simulink model "WaterTankSysControlPID2024"  (R2023b)
settings: Solver=FixedStepAuto  StartTime=0.0  StopTime=525  FixedStep=0.75  RelTol=1e-3  EnableMultiTasking=on
StopFcn:
  | FileName='PIDControlData0.mat';
  | [fPath, fName, fExt] = fileparts(FileName);
  | if isempty(fExt)  % No '.mat' in FileName
  |     fExt     = '.mat';
  |     FileName = fullfile(fPath, [fName, fExt]);
  | end
  | if exist(FileName, 'file')
  |     % Get number of files:
  |     fDir     = dir(fullfile(fPath, [fName, '*', fExt]));
  |     fStr     = lower(sprintf('%s*', fDir.name));
  |     %fNum     = sscanf(fStr, [fName, '%d', fExt, '*']);
  |     digit =  str2double(extract(fStr, digitsPattern));
  |     %newNum = digit + 1;
  |     if isempty(digit)
  |         newNum = 1;
  |     else
  |         newNum = digit + 1;
  |     end
  |     FileName = fullfile(fPath, [fName, sprintf('%d', newNum(end)), fExt]);
  | end
  | save(FileName, 'ScopeData1');
  | clear digit fDir fExt FileName fName fPath fStr newNum fNum
values from neighbouring files (symbols this model uses):
  u_offset = u_act(1)    [Lab5.m]
  y_offset = mean(y_act(1:i))    [Lab5.m]
undefined symbols (not defined in the file or in its folder): National_Instruments, PCIe
libraries: sldrtlib x4, slpidlib x1, simulink x1
settings Model: SimulationMode=external  ExtModeTrigDuration=7200  ExtModeArchiveMode=auto  ExtModeArchiveFileName=SysIdenData  ExtModeArchiveDirName=C:\Users\My Project\Documents\MATLAB  ExtModeAutoIncOneShot=on  ExtModeWriteAllDataToWs=on  Creator=My Project  LastModifiedBy=My Project
settings SolverCC: AlgebraicLoopSolver=TrustRegion
settings DataIOCC: LimitDataPoints=on  ReturnWorkspaceOutputs=off
settings OptimizationCC: ReuseModelBlockBuffer=off  LifeSpan=inf
settings DebuggingCC: UnconnectedInputMsg=warning  UnconnectedOutputMsg=warning  UnconnectedLineMsg=warning  AllowSymbolicDim=off  SFUnexpectedBacktrackingDiag=warning  SFNoUnconditionalDefaultTransitionDiag=warning  SFExecutionAtInitializationDiag=none  ArithmeticOperatorsInVariantConditions=warning
settings HardwareCC: ProdBitPerLong=64  ProdHWDeviceType=Intel->x86-64 (Linux 64)  TargetBitPerLong=64  TargetBitPerPointer=64  TargetIntDivRoundTo=Zero  TargetEndianess=LittleEndian  TargetWordSize=64  TargetHWDeviceType=Intel->x86-64
settings ModelReferenceCC: EnableRefExpFcnMdlSchedulingChecks=on  PropagateSignalLabelsOutOfModel=off
settings SFSimCC: SimUseLocalCustomCode=off  CustomCodeUndefinedFunction=UseInterfaceOnly
settings RTWCC: Description=Simulink Desktop Real-Time  SystemTargetFile=sldrt.tlc  TemplateMakefile=sldrt.tmf  RTWUseLocalCustomCode=off  RTWCompilerOptimization=on
settings CodeAppCC: MaxIdLength=95  StateflowObjectComments=on
settings SimulinkDesktopRealTimeCC: TargetLibSuffix=_sldrt.a  TargetPreCompLibLocation=C:\Program Files\MATLAB\R2023b\toolbox\sldrt\lib\win64  TargetLangStandard=C89/C90 (ANSI)  SupportVariableSizeSignals=off
settings ConfigComp: CovMetricSettings=dw  CovSaveCumulativeToWorkspaceVar=on  CovSaveSingleToWorkspaceVar=on  CovExternalEMLEnable=off

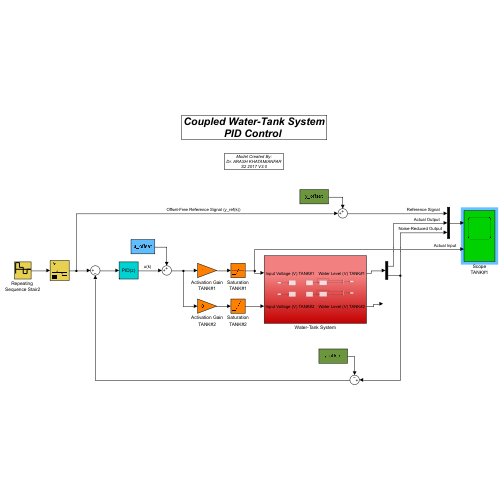
[thumbnail: Simulink's stored preview of the top-level diagram]
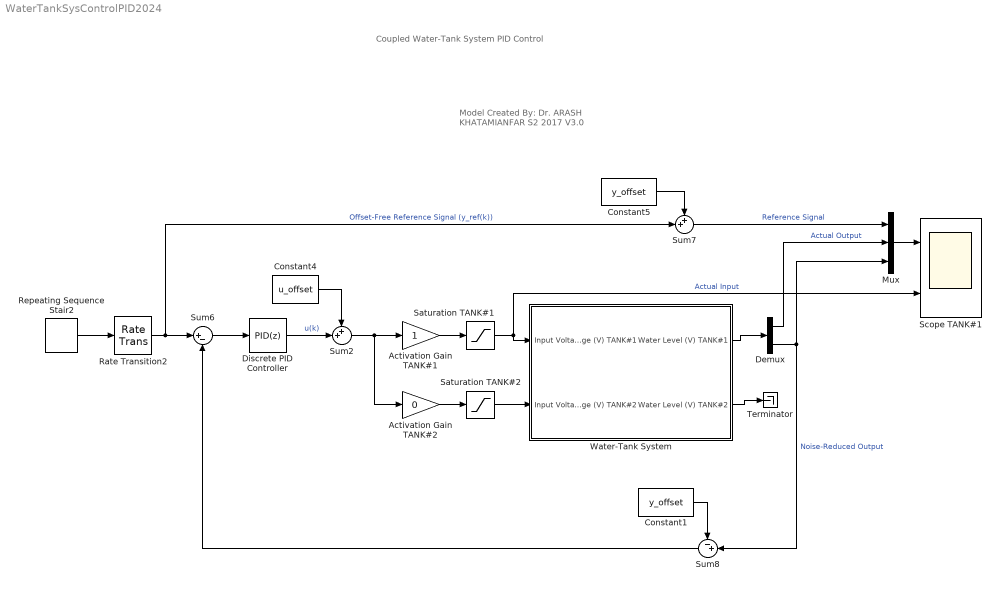
== system WaterTankSysControlPID2024 ==
  note: Model Created By:
      | Dr. ARASH KHATAMIANFAR
      | S2 2017 V3.0
  note: Coupled Water-Tank System
      | PID Control
  Activation Gain TANK#1 : Gain
  Activation Gain TANK#2 : Gain  Gain=0
  Constant1 : Constant  Value=y_offset
  Constant4 : Constant  Value=u_offset
  Constant5 : Constant  Value=y_offset
  Demux : Demux  Outputs=2
  Discrete PID Controller : slpidlib/PID Controller  Controller=PID  Form=Parallel  TimeDomain=Discrete-time  UseExternalTs=off  SampleTime=0.75  IntegratorMethod=Forward Euler  FilterMethod=Forward Euler  ControllerParametersSource=internal  P=0.56  I=0.029  UseKiTs=off  D=0  N=100  UseFilter=on  TunerSelectOption=Transfer Function Based (PID Tuner App)  InitialConditionSource=internal  InitialConditionForIntegrator=0  InitialConditionForFilter=0  DifferentiatorICPrevScaledInput=0  ExternalReset=none  TrackingMode=off  Kt=1  LimitOutput=off  SatLimitsSource=internal  UpperSaturationLimit=inf  LowerSaturationLimit=-inf  LinearizeAsGain=off  AntiWindupMode=none  Kb=1  LimitIntegrator=off  UpperIntegratorSaturationLimit=1  LowerIntegratorSaturationLimit=-1  POutMin=[]  POutMax=[]  IOutMin=[]  IOutMax=[]  DOutMin=[]  DOutMax=[]  NOutMin=[]  NOutMax=[]  SumOutMin=[]  SumOutMax=[]  SaturationOutMin=[]  SaturationOutMax=[]  PParamMin=[]  PParamMax=[]  IParamMin=[]  IParamMax=[]  DParamMin=[]  DParamMax=[]  NParamMin=[]  NParamMax=[]  KbParamMin=[]  KbParamMax=[]  KtParamMin=[]  KtParamMax=[]  KbOutMin=[]  KbOutMax=[]  KtOutMin=[]  KtOutMax=[]  IntegratorOutMin=[]  IntegratorOutMax=[]  FilterOutMin=[]  FilterOutMax=[]  SumI1OutMin=[]  SumI1OutMax=[]  SumI2OutMin=[]  SumI2OutMax=[]  SumI3OutMin=[]  SumI3OutMax=[]  SumI4OutMin=[]  SumI4OutMax=[]  SumDOutMin=[]  SumDOutMax=[]  DifferentiatorOutMin=[]  DifferentiatorOutMax=[]  FilterDiffOutCoefMin=[]  FilterDiffOutCoefMax=[]  ReciprocalOutMin=[]  ReciprocalOutMax=[]  SumDenOutMin=[]  SumDenOutMax=[]  SumNumOutMin=[]  SumNumOutMax=[]  DivideOutMin=[]  DivideOutMax=[]  UdiffTsProdOutMin=[]  UdiffTsProdOutMax=[]  NTsProdOutMin=[]  NTsProdOutMax=[]  UintegralTsProdOutMin=[]  UintegralTsProdOutMax=[]  UngainTsProdOutMin=[]  UngainTsProdOutMax=[]  ClampingZeroOutDataTypeStr=Inherit: Inherit via back propagation  ClampingZeroOutMin=[]  ClampingZeroOutMax=[]  FilterDenConstantOutDataTypeStr=Inherit: Inherit via back propagation  FilterDenConstantOutMin=[]  FilterDenConstantOutMax=[]  PCopyOutDataTypeStr=Inherit: Inherit via back propagation  PCopyOutMin=[]  PCopyOutMax=[]  NCopyOutDataTypeStr=Inherit: Inherit via back propagation  NCopyOutMin=[]  NCopyOutMax=[]  IntegratorContinuousStateAttributes=''  IntegratorStateMustResolveToSignalObject=off  IntegratorRTWStateStorageClass=Auto  FilterContinuousStateAttributes=''  FilterStateMustResolveToSignalObject=off  FilterRTWStateStorageClass=Auto  ParallelPVariant=InternalParameters  IdealPVariant=Disabled  IVariant=InternalParameters  DVariant=InternalParameters  IntegratorVariant=Discrete  SatVariant=Disabled  AWVariant=Passthrough  PCopyVariant=Disabled  TRVariant=Disabled  FdbkBlocksVariant=Forward  IdealPFdbkVariant=Disabled  SatFdbkVariant=Disabled  DerivativeFilterVariant=ForwardEulerFilter  NVariant=InternalParameters  NCopyVariant=Disabled  FilterICVariant=InternalICsFilter  IntegratorICVariant=InternalICs  ExternalResetVariant=Disabled  TRSumVariant=Passthrough  SumFdbkVariant=Disabled  SumVariant=Sum_PID  TsampFilterVariant=InternalTs  TsampNgainVariant=Passthrough  TsampIntegralVariant=Disabled_SignalSpec  ExternalSaturationOutDataTypeStr=Inherit: Same as second input
  Mux : Mux  Inputs=3
  Rate Transition2 : RateTransition  OutPortSampleTime=0.75
  Repeating Sequence Stair2 : simulink/Sources/Repeating Sequence Stair  OutValues=[ 0.7 0.2 -0.5 0].'  tsamp=140*0.75  OutMin=[]  OutMax=[]  OutDataTypeStr=double  OutputDataTypeScalingMode=double  OutDataType=fixdt(0,8)  ConRadixGroup=Best Precision: Vector-wise  OutScaling=2^-12
  Saturation TANK#1 : Saturate  UpperLimit=3  LowerLimit=2
  Saturation TANK#2 : Saturate  UpperLimit=5  LowerLimit=0
  Scope TANK#1 : Scope  NumInputPorts=2
  Sum2 : Sum  Inputs=++|
  Sum6 : Sum  Inputs=|+-
  Sum7 : Sum  Inputs=++|
  Sum8 : Sum  Inputs=-+|
  Terminator : Terminator
  Water-Tank System : Subsystem
  wires:
  Sum7/1 -> Mux/1  "Reference Signal"
  Water-Tank System/1(Water Level (V) TANK#1) -> Demux/1
  Discrete PID Controller/1 -> Sum2/2  "u(k)"
  Saturation TANK#1/1 -> Scope TANK#1/2, Water-Tank System/1(Input Voltage (V) TANK#1)  "Actual Input"
  Sum2/1 -> Activation Gain TANK#2/1, Activation Gain TANK#1/1
  Sum8/1 -> Sum6/2
  Constant1/1 -> Sum8/1
  Demux/2 -> Sum8/2, Mux/3  "Noise-Reduced Output"
  Demux/1 -> Mux/2  "Actual Output"
  Saturation TANK#2/1 -> Water-Tank System/2(Input Voltage (V) TANK#2)
  Mux/1 -> Scope TANK#1/1
  Activation Gain TANK#2/1 -> Saturation TANK#2/1
  Constant5/1 -> Sum7/1
  Repeating Sequence Stair2/1 -> Rate Transition2/1
  Constant4/1 -> Sum2/1
  Activation Gain TANK#1/1 -> Saturation TANK#1/1
  Sum6/1 -> Discrete PID Controller/1
  Water-Tank System/2(Water Level (V) TANK#2) -> Terminator/1
  Rate Transition2/1 -> Sum6/1, Sum7/2  "Offset-Free Reference Signal (y_ref(k))"

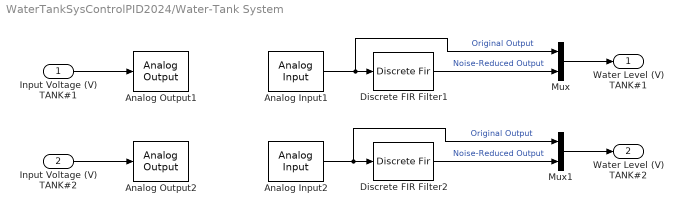
== system WaterTankSysControlPID2024/Water-Tank System ==
  Input Voltage (V) TANK#1 : Inport
  Input Voltage (V) TANK#2 : Inport  Port=2
  Analog Input1 : sldrtlib/Analog Input  SampleTime=0.75  MaxMissedTicks=10  ShowMissedTicks=off  YieldWhenWaiting=off  DrvName=National_Instruments/PCIe-6351  DrvAddress=4294967295  DrvOptions=[0 0 0 0 0 0 0]  Channels=1  RangeMode=1  VoltRange=1  DataType=1
      settings: AttributesFormatString=National Instruments\nPCIe-6351 [auto]
  Analog Input2 : sldrtlib/Analog Input  SampleTime=0.75  MaxMissedTicks=10  ShowMissedTicks=off  YieldWhenWaiting=off  DrvName=National_Instruments/PCIe-6351  DrvAddress=4294967295  DrvOptions=[0 0 0 0 0 0 0]  Channels=2  RangeMode=1  VoltRange=1  DataType=1
      settings: AttributesFormatString=National Instruments\nPCIe-6351 [auto]
  Analog Output1 : sldrtlib/Analog Output  SampleTime=0.75  MaxMissedTicks=10  ShowMissedTicks=off  YieldWhenWaiting=off  DrvName=National_Instruments/PCIe-6351  DrvAddress=4294967295  DrvOptions=[0 0 0 0 0 0 0]  Channels=1  RangeMode=1  VoltRange=1  InitialValue=0  FinalValue=0
      settings: AttributesFormatString=National Instruments\nPCIe-6351 [auto]
  Analog Output2 : sldrtlib/Analog Output  SampleTime=0.75  MaxMissedTicks=10  ShowMissedTicks=off  YieldWhenWaiting=off  DrvName=National_Instruments/PCIe-6351  DrvAddress=4294967295  DrvOptions=[0 0 0 0 0 0 0]  Channels=2  RangeMode=1  VoltRange=1  InitialValue=0  FinalValue=0
      settings: AttributesFormatString=National Instruments\nPCIe-6351 [auto]
  Discrete FIR Filter1 : DiscreteFir  Coefficients=[0.2 0.2 0.2 0.2 0.2]  SampleTime=0.75
  Discrete FIR Filter2 : DiscreteFir  Coefficients=[0.2 0.2 0.2 0.2 0.2]  SampleTime=0.75
  Mux : Mux  Inputs=2
  Mux1 : Mux  Inputs=2
  Water Level (V) TANK#1 : Outport
  Water Level (V) TANK#2 : Outport  Port=2
  wires:
  Analog Input1/1 -> Mux/1, Discrete FIR Filter1/1  "Original Output"
  Input Voltage (V) TANK#1/1 -> Analog Output1/1
  Discrete FIR Filter1/1 -> Mux/2  "Noise-Reduced Output"
  Mux/1 -> Water Level (V) TANK#1/1
  Analog Input2/1 -> Mux1/1, Discrete FIR Filter2/1  "Original Output"
  Input Voltage (V) TANK#2/1 -> Analog Output2/1
  Discrete FIR Filter2/1 -> Mux1/2  "Noise-Reduced Output"
  Mux1/1 -> Water Level (V) TANK#2/1
